simulink model "sim_control_pd_g_2DOF"  (R2019b)
settings: Solver=VariableStepAuto  StartTime=0.0  StopTime=10.0  RelTol=1e-3
values from neighbouring files (symbols this model uses):
  Kd = [Kp1*Td1 0;         0       Kp2*Td2]    [control_pd_g.m]
  Kp = [Kp1 0;         0   Kp2]    [control_pd_g.m]
  q0 = [90*pi/180;0;0;0]    [control_pd_g.m]
  q_ = [110*pi/180;-30*pi/180;0;0]    [control_pd_g.m]
  theta = load('../theta.mat').theta    [control_pd_g.m]    (also in modelo_dinamico_lineal.m)
settings Model: Creator=AlejnadroZapett  LastModifiedBy=AlejnadroZapett

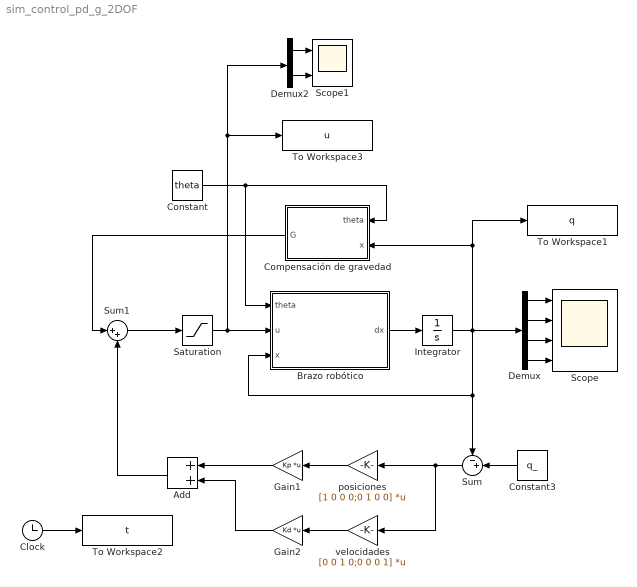
== system sim_control_pd_g_2DOF ==
  Add : Sum
  Brazo robótico : MATLAB Function  TreatAsAtomicUnit=on
  Clock : Clock
  Compensación de gravedad : MATLAB Function  TreatAsAtomicUnit=on
  Constant : Constant  Value=theta
  Constant3 : Constant  Value=q_
  Demux : Demux
  Demux2 : Demux  Outputs=2
  Gain1 : Gain  Gain=Kp  Multiplication=Matrix(K*u) (u vector)
  Gain2 : Gain  Gain=Kd  Multiplication=Matrix(K*u) (u vector)
  Integrator : Integrator  InitialCondition=q0
  Saturation : Saturate  UpperLimit=255  LowerLimit=-255
  Scope : Scope  NumInputPorts=4
  Scope1 : Scope  NumInputPorts=2
  Sum : Sum  Inputs=-+|
  Sum1 : Sum  Inputs=|++
  To Workspace1 : ToWorkspace  VariableName=q  SampleTime=-1
  To Workspace2 : ToWorkspace  VariableName=t  SampleTime=-1
  To Workspace3 : ToWorkspace  VariableName=u  SampleTime=-1
  posiciones : Gain  Gain=[1 0 0 0;0 1 0 0]  Multiplication=Matrix(K*u) (u vector)
  "velocidades " : Gain  Gain=[0 0 1 0;0 0 0 1]  Multiplication=Matrix(K*u) (u vector)
  wires:
  Demux/4 -> Scope/4
  Demux2/2 -> Scope1/2
  Integrator/1 -> Compensación de gravedad/2(x), To Workspace1/1, Demux/1, Sum/1, Brazo robótico/3(x)
  Constant/1 -> Compensación de gravedad/1(theta), Brazo robótico/1(theta)
  Demux/1 -> Scope/1
  Brazo robótico/1(dx) -> Integrator/1
  Demux/2 -> Scope/2
  Demux/3 -> Scope/3
  Demux2/1 -> Scope1/1
  Clock/1 -> To Workspace2/1
  Sum1/1 -> Saturation/1
  Saturation/1 -> Brazo robótico/2(u), To Workspace3/1, Demux2/1
  posiciones/1 -> Gain1/1
  "velocidades "/1 -> Gain2/1
  Gain1/1 -> Add/1
  Gain2/1 -> Add/2
  Constant3/1 -> Sum/2
  Sum/1 -> "velocidades "/1, posiciones/1
  Add/1 -> Sum1/2
  Compensación de gravedad/1(G) -> Sum1/1

== matlab function sim_control_pd_g_2DOF/Compensación de gravedad ==
  data: theta input; G output; x input
function G = fcn(theta,x)

q1 = x(1);
q2 = x(2);

G1 = theta(7)*cos(q1)+theta(8)*cos(q1+q2);
G2 = theta(14)*cos(q1+q2);

G = [G1;G2];

== matlab function sim_control_pd_g_2DOF/Brazo robótico ==
  data: theta input; u input; dx output; x input
function dx = fcn(theta,u,x)

dx = zeros(4,1);

u1 = u(1);
u2 = u(2);

q1 = x(1);
q2 = x(2);
dq1 = x(3);
dq2 = x(4);

M11 = (theta(1) + theta(2)*cos(q1));
M12 = (theta(3) + theta(4)*cos(q2));
M21 = (theta(11) + theta(12)*cos(q2));
M22 = theta(13);

C11 = theta(5)*sin(q2)*dq2;
C12 = theta(6)*sin(q2)*dq2;
C21 = theta(14)*sin(q2)*dq1;
C22 = 0;

G1 = theta(7)*cos(q1)+theta(8)*cos(q1+q2);
G2 = theta(14)*cos(q1+q2);

% F1 = theta(9)*dq1 + theta(10)*sign(dq1);
% F2 = theta(16)*dq2 + theta(17)*sign(dq2);
F1 = theta(9)*dq1;
F2 = theta(16)*dq2;

M = [M11 M12;M21 M22];
C = [C11 C12;C21 C22];
G = [G1;G2];
F = [F1;F2];
T = [u1;u2];

D = -inv(M)*(C*[dq1;dq2]+G+F-T);

dx(1) = dq1;
dx(2) = dq2;
dx(3) = D(1);
dx(4) = D(2);
